simulink model "system_using_controller_design"  (R2021a)
settings: Solver=VariableStepAuto  StartTime=0.0  StopTime=1  RelTol=1e-3
values from neighbouring files (symbols this model uses):
  A = [0 0 1 0;0 0 0 1;1 0 0 -20;4.998 -70 -49.98 0]    [Controlib.m]    (also in Observ.m = [0 0 1 0; 0 0 0 1;1 0 0 -20;4.998 -70 -49.98 0]; Opp.m = double(subs(jac,[x1,x2,x3,x4],[op1,op2,op3,op4])); Stabili.m = [0 0 1 0; 0 0 0 1;1 0 0 -20;4.998 -70 -49.98 0]; lyaptesting.m = [0 0 1 0;0 0 0 1;1 0 0 -20;5 -70 -50 0])
  B = [0 0;0 0;F/7 0;0 M/2]    [Controlib.m]    (also in Linearization.m; Observ.m = [0 0;0 0 ;F/7 0 ; 0 M/2]; Opp.m; Stabili.m = [0 0;0 0; F/7 0; 0 M/2])
  K = place(A,B,PR)    [Poleplace.m]
settings Model: Creator=Musthafa  LastModifiedBy=Musthafa

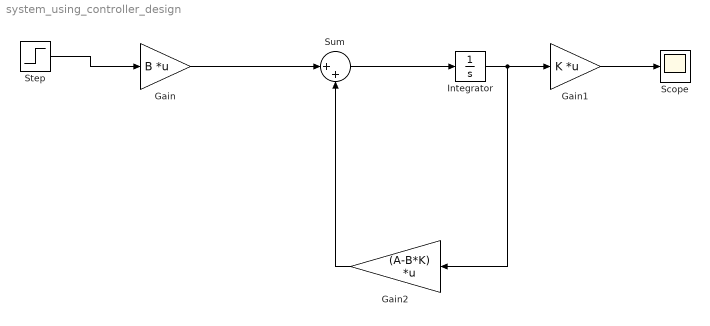
== system system_using_controller_design ==
  Gain : Gain  Gain=B  Multiplication=Matrix(K*u) (u vector)
  Gain1 : Gain  Gain=K  Multiplication=Matrix(K*u) (u vector)
  Gain2 : Gain  Gain=(A-B*K)  Multiplication=Matrix(K*u) (u vector)
  Integrator : Integrator
  Scope : Scope
  Step : Step  SampleTime=0
  Sum : Sum  Inputs=|++
  wires:
  Gain2/1 -> Sum/2
  Step/1 -> Gain/1
  Gain/1 -> Sum/1
  Sum/1 -> Integrator/1
  Integrator/1 -> Gain2/1, Gain1/1
  Gain1/1 -> Scope/1
